simulink model "ActiveBalancerCopy"  (R2021a)
settings: Solver=VariableStepAuto  StartTime=0.0  StopTime=30  RelTol=1e-3
undefined symbols (not defined in the file): Ion, Lithium
libraries: spsIdealSwitchLib x12, spsSeriesRLCBranchLib x12, spsBatteryLib x6, spsDiodeLib x6, spsDCVoltageSourceLib x3, spsGroundLib x3, spsPWMGenerator2LevelLib x3, spspowerguiLib x1
settings Model: Creator=jafar  LastModifiedBy=jafar

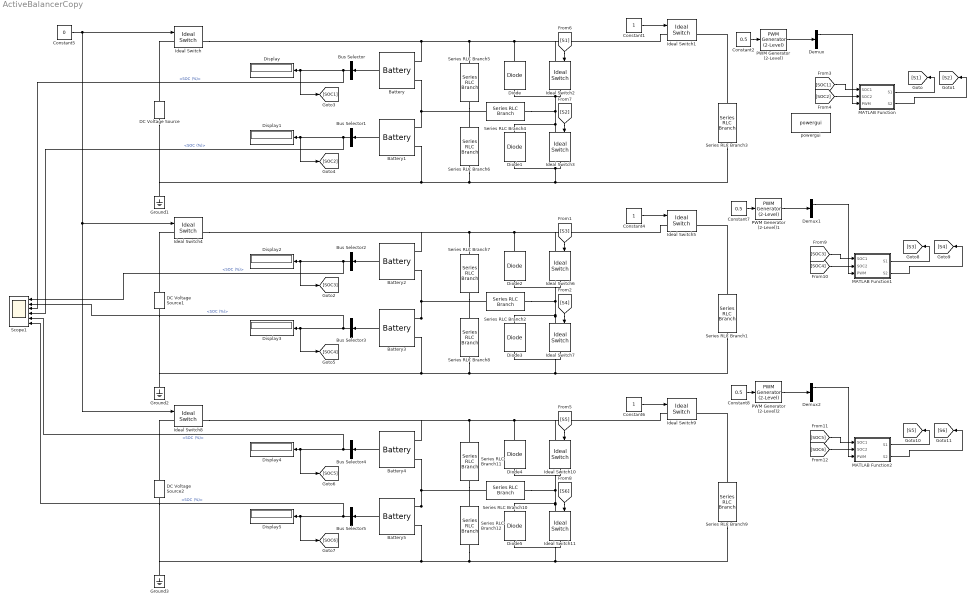
== system ActiveBalancerCopy ==
  Battery : spsBatteryLib/Battery  BatType=Lithium-Ion  ShowTempParam=off  ThermalPreset=no  ShowAgeParam=off  NomV=3.7  NomQ=5.4  SOC=20  Batt_Tr=30  PresetModel=on  MaxQ=5.4  MinV=2.775  FullV=4.3068  Dis_rate=2.3478  R=0.0068519  Normal_OP=4.8835  expZone="[3.9974      0.2653]"  current=[6.5 13 32.5]  Units=Time  Tci=20  NomT=20  T2=-30  MaxQ2=4.8  FullV2=7.1  Normal_OP2=5.655  expZone2="[6.58           1]"  Rca=0.6  ti=2000  Dp=0  Neq0=0  Tsim=1e6  Ta1=25  Qeol=5.4*0.9  Reol=0.013333*1.2  Char_age=[2.3478, 3]  Dis_age=[2.3478, 10]  N1=1500  N2=10500  N3=1000  N4=1400  Ta2=45  N5=950
  Battery1 : spsBatteryLib/Battery  BatType=Lithium-Ion  ShowTempParam=off  ThermalPreset=no  ShowAgeParam=off  NomV=3.7  NomQ=5.4  SOC=30  Batt_Tr=30  PresetModel=on  MaxQ=5.4  MinV=2.775  FullV=4.3068  Dis_rate=2.3478  R=0.0068519  Normal_OP=4.8835  expZone="[3.9974      0.2653]"  current=[6.5 13 32.5]  Units=Time  Tci=20  NomT=20  T2=-30  MaxQ2=4.8  FullV2=7.1  Normal_OP2=5.655  expZone2="[6.58           1]"  Rca=0.6  ti=2000  Dp=0  Neq0=0  Tsim=1e6  Ta1=25  Qeol=5.4*0.9  Reol=0.013333*1.2  Char_age=[2.3478, 3]  Dis_age=[2.3478, 10]  N1=1500  N2=10500  N3=1000  N4=1400  Ta2=45  N5=950
  Battery2 : spsBatteryLib/Battery  BatType=Lithium-Ion  ShowTempParam=off  ThermalPreset=no  ShowAgeParam=off  NomV=3.7  NomQ=5.4  SOC=40  Batt_Tr=30  PresetModel=on  MaxQ=5.4  MinV=2.775  FullV=4.3068  Dis_rate=2.3478  R=0.0068519  Normal_OP=4.8835  expZone="[3.9974      0.2653]"  current=[6.5 13 32.5]  Units=Time  Tci=20  NomT=20  T2=-30  MaxQ2=4.8  FullV2=7.1  Normal_OP2=5.655  expZone2="[6.58           1]"  Rca=0.6  ti=2000  Dp=0  Neq0=0  Tsim=1e6  Ta1=25  Qeol=5.4*0.9  Reol=0.013333*1.2  Char_age=[2.3478, 3]  Dis_age=[2.3478, 10]  N1=1500  N2=10500  N3=1000  N4=1400  Ta2=45  N5=950
  Battery3 : spsBatteryLib/Battery  BatType=Lithium-Ion  ShowTempParam=off  ThermalPreset=no  ShowAgeParam=off  NomV=3.7  NomQ=5.4  SOC=50  Batt_Tr=30  PresetModel=on  MaxQ=5.4  MinV=2.775  FullV=4.3068  Dis_rate=2.3478  R=0.0068519  Normal_OP=4.8835  expZone="[3.9974      0.2653]"  current=[6.5 13 32.5]  Units=Time  Tci=20  NomT=20  T2=-30  MaxQ2=4.8  FullV2=7.1  Normal_OP2=5.655  expZone2="[6.58           1]"  Rca=0.6  ti=2000  Dp=0  Neq0=0  Tsim=1e6  Ta1=25  Qeol=5.4*0.9  Reol=0.013333*1.2  Char_age=[2.3478, 3]  Dis_age=[2.3478, 10]  N1=1500  N2=10500  N3=1000  N4=1400  Ta2=45  N5=950
  Battery4 : spsBatteryLib/Battery  BatType=Lithium-Ion  ShowTempParam=off  ThermalPreset=no  ShowAgeParam=off  NomV=3.7  NomQ=5.4  SOC=60  Batt_Tr=30  PresetModel=on  MaxQ=5.4  MinV=2.775  FullV=4.3068  Dis_rate=2.3478  R=0.0068519  Normal_OP=4.8835  expZone="[3.9974      0.2653]"  current=[6.5 13 32.5]  Units=Time  Tci=20  NomT=20  T2=-30  MaxQ2=4.8  FullV2=7.1  Normal_OP2=5.655  expZone2="[6.58           1]"  Rca=0.6  ti=2000  Dp=0  Neq0=0  Tsim=1e6  Ta1=25  Qeol=5.4*0.9  Reol=0.013333*1.2  Char_age=[2.3478, 3]  Dis_age=[2.3478, 10]  N1=1500  N2=10500  N3=1000  N4=1400  Ta2=45  N5=950
  Battery5 : spsBatteryLib/Battery  BatType=Lithium-Ion  ShowTempParam=off  ThermalPreset=no  ShowAgeParam=off  NomV=3.7  NomQ=5.4  SOC=70  Batt_Tr=30  PresetModel=on  MaxQ=5.4  MinV=2.775  FullV=4.3068  Dis_rate=2.3478  R=0.0068519  Normal_OP=4.8835  expZone="[3.9974      0.2653]"  current=[6.5 13 32.5]  Units=Time  Tci=20  NomT=20  T2=-30  MaxQ2=4.8  FullV2=7.1  Normal_OP2=5.655  expZone2="[6.58           1]"  Rca=0.6  ti=2000  Dp=0  Neq0=0  Tsim=1e6  Ta1=25  Qeol=5.4*0.9  Reol=0.013333*1.2  Char_age=[2.3478, 3]  Dis_age=[2.3478, 10]  N1=1500  N2=10500  N3=1000  N4=1400  Ta2=45  N5=950
  Bus Selector{,1..5} (6 alike) : BusSelector  OutputSignals=SOC (%)
  Constant1 : Constant
  Constant2 : Constant  Value=0.5
  Constant4 : Constant
  Constant5 : Constant  Value=0
  Constant6 : Constant
  Constant7 : Constant  Value=0.5
  Constant8 : Constant  Value=0.5
  DC Voltage Source : spsDCVoltageSourceLib/DC Voltage Source  Amplitude=12  Measurements=None
  DC Voltage Source1 : spsDCVoltageSourceLib/DC Voltage Source  Amplitude=12  Measurements=None
  DC Voltage Source2 : spsDCVoltageSourceLib/DC Voltage Source  Amplitude=12  Measurements=None
  Demux : Demux  Outputs=2
  Demux1 : Demux  Outputs=2
  Demux2 : Demux  Outputs=2
  Diode{,1..5} (6 alike) : spsDiodeLib/Diode  Ron=0.001  Lon=0  Vf=0.8  IC=0  UseSnubber=0  Rs=500  Cs=250e-9  Measurements=off
  Display{,1..5} (6 alike) : Display
  Ground1 : spsGroundLib/Ground  LConnTagsString=a
  Ground2 : spsGroundLib/Ground  LConnTagsString=a
  Ground3 : spsGroundLib/Ground  LConnTagsString=a
  Ideal Switch{,1,4..5,8..9} (6 alike) : spsIdealSwitchLib/Ideal Switch  Ron=0.001  Lon=0  IC=0  Rs=1e5  Cs=inf  Measurements=on
  Ideal Switch{2..3,6..7,10..11} (6 alike) : spsIdealSwitchLib/Ideal Switch  Ron=0.001  Lon=0  IC=0  Rs=1e5  Cs=inf  Measurements=off
  MATLAB Function : MATLAB Function  TreatAsAtomicUnit=on
  MATLAB Function1 : MATLAB Function  TreatAsAtomicUnit=on
  MATLAB Function2 : MATLAB Function  TreatAsAtomicUnit=on
  PWM Generator (2-Level) : spsPWMGenerator2LevelLib/PWM Generator (2-Level)  ModulatorType=Single-phase half-bridge (2 pulses)  ModulatorMode=Unsynchronized  Fc=500  Pc=0  nF=27  MinMax="[ -1  1 ]"  SamplingTechnique=Natural  ModulatingSignals=off  m=0.8  Freq=60  Phase=0  Ts=0  ShowCarrierOutport=off
  PWM Generator (2-Level)1 : spsPWMGenerator2LevelLib/PWM Generator (2-Level)  ModulatorType=Single-phase half-bridge (2 pulses)  ModulatorMode=Unsynchronized  Fc=500  Pc=0  nF=27  MinMax="[ -1  1 ]"  SamplingTechnique=Natural  ModulatingSignals=off  m=0.8  Freq=60  Phase=0  Ts=0  ShowCarrierOutport=off
  PWM Generator (2-Level)2 : spsPWMGenerator2LevelLib/PWM Generator (2-Level)  ModulatorType=Single-phase half-bridge (2 pulses)  ModulatorMode=Unsynchronized  Fc=500  Pc=0  nF=27  MinMax="[ -1  1 ]"  SamplingTechnique=Natural  ModulatingSignals=off  m=0.8  Freq=60  Phase=0  Ts=0  ShowCarrierOutport=off
  Scope1 : Scope  NumInputPorts=6
  Series RLC Branch1 : spsSeriesRLCBranchLib/Series RLC Branch  LConnTagsString=__new0  RConnTagsString=__new0  BranchType=R  Resistance=1  Inductance=1e-3  SetiL0=off  InitialCurrent=0  Capacitance=1e-6  Setx0=off  InitialVoltage=0  Measurements=None
  Series RLC Branch10 : spsSeriesRLCBranchLib/Series RLC Branch  LConnTagsString=__new0  RConnTagsString=__new0  BranchType=L  Resistance=1  Inductance=1e-3  SetiL0=off  InitialCurrent=0  Capacitance=1e-6  Setx0=off  InitialVoltage=0  Measurements=None
  Series RLC Branch{5..8,11..12} (6 alike) : spsSeriesRLCBranchLib/Series RLC Branch  LConnTagsString=__new0  RConnTagsString=__new0  BranchType=C  Resistance=1  Inductance=1e-3  SetiL0=off  InitialCurrent=0  Capacitance=1e-6  Setx0=off  InitialVoltage=0  Measurements=None
  Series RLC Branch2 : spsSeriesRLCBranchLib/Series RLC Branch  LConnTagsString=__new0  RConnTagsString=__new0  BranchType=L  Resistance=1  Inductance=1e-3  SetiL0=off  InitialCurrent=0  Capacitance=1e-6  Setx0=off  InitialVoltage=0  Measurements=None
  Series RLC Branch3 : spsSeriesRLCBranchLib/Series RLC Branch  LConnTagsString=__new0  RConnTagsString=__new0  BranchType=R  Resistance=1  Inductance=1e-3  SetiL0=off  InitialCurrent=0  Capacitance=1e-6  Setx0=off  InitialVoltage=0  Measurements=None
  Series RLC Branch4 : spsSeriesRLCBranchLib/Series RLC Branch  LConnTagsString=__new0  RConnTagsString=__new0  BranchType=L  Resistance=1  Inductance=1e-3  SetiL0=off  InitialCurrent=0  Capacitance=1e-6  Setx0=off  InitialVoltage=0  Measurements=None
  Series RLC Branch9 : spsSeriesRLCBranchLib/Series RLC Branch  LConnTagsString=__new0  RConnTagsString=__new0  BranchType=R  Resistance=1  Inductance=1e-3  SetiL0=off  InitialCurrent=0  Capacitance=1e-6  Setx0=off  InitialVoltage=0  Measurements=None
  powergui : spspowerguiLib/powergui  Priority=1  SimulationMode=Discrete  SampleTime=50e-5  frequency=60  Iterations=50  frequencyindice=0  Pbase=100e6  ErrMax=1e-4  UnitsV=kV  UnitsW=MW  buscounter=0  FunctionMessages=off  echomessages=off  EnableUseOfTLC=off  CurrentSourceSwitches=off  DisableSnubberDevices=off  DisableRonSwitches=off  DisableVfSwitches=off  DisplayEquations=off  AutomaticDiscreteSolvers=off  SolverType=Tustin/Backward Euler (TBE)  Interpol=off  ExternalGateDelay=off  methode=off  Ts=100  x0status=blocks  SPID=on  SwTol=0  HookPort=off  NonlinearTolerance=1e-4  nMaxIteration=100  ContinueOnMaxIteration=off  RestoreLinks=warning  ResistiveCurrentMeasurement=off  Frange=[0:2:500]  Ylog=off  Xlog=on  ShowGrid=off  save=off  variable=ZData  structure=0  ZoomFFT=off  StartTime=0.0  cycles=1  DisplayStyle=1  fundamental=60  FreqAxis=off  MaxFrequency=1000  frequencyindicesteady=1  RmsSteady=1  display=off
  wires:
  [SOC1] -> MATLAB Function/1(SOC1)
  [SOC2] -> MATLAB Function/2(SOC2)
  Constant5/1 -> Ideal Switch/1, Ideal Switch4/1, Ideal Switch8/1
  MATLAB Function/1(S1) -> [S1]
  Battery/1 -> Bus Selector/1
  Bus Selector1/1 -> Scope1/4, [SOC2], Display1/1  "<SOC (%)>"
  Battery1/1 -> Bus Selector1/1
  MATLAB Function/2(S2) -> [S2]
  Constant1/1 -> Ideal Switch1/1
  Bus Selector/1 -> Scope1/3, [SOC1], Display/1  "<SOC (%)>"
  [S1] -> Ideal Switch2/1
  [S2] -> Ideal Switch3/1
  Constant2/1 -> PWM Generator (2-Level)/1
  PWM Generator (2-Level)/1 -> Demux/1
  Demux/1 -> MATLAB Function/3(PWM)
  Battery3/1 -> Bus Selector3/1
  Bus Selector3/1 -> Scope1/2, [SOC4], Display3/1  "<SOC (%)>"
  Bus Selector2/1 -> Scope1/1, [SOC3], Display2/1  "<SOC (%)>"
  [S3] -> Ideal Switch6/1
  [S4] -> Ideal Switch7/1
  Battery2/1 -> Bus Selector2/1
  Constant4/1 -> Ideal Switch5/1
  Battery5/1 -> Bus Selector5/1
  Bus Selector5/1 -> Scope1/6, [SOC6], Display5/1  "<SOC (%)>"
  Bus Selector4/1 -> Scope1/5, [SOC5], Display4/1  "<SOC (%)>"
  [S5] -> Ideal Switch10/1
  [S6] -> Ideal Switch11/1
  Battery4/1 -> Bus Selector4/1
  Constant6/1 -> Ideal Switch9/1
  Constant7/1 -> PWM Generator (2-Level)1/1
  Demux1/1 -> MATLAB Function1/3(PWM)
  [SOC4] -> MATLAB Function1/2(SOC2)
  MATLAB Function1/2(S2) -> [S4]
  MATLAB Function1/1(S1) -> [S3]
  PWM Generator (2-Level)1/1 -> Demux1/1
  [SOC3] -> MATLAB Function1/1(SOC1)
  Constant8/1 -> PWM Generator (2-Level)2/1
  Demux2/1 -> MATLAB Function2/3(PWM)
  [SOC6] -> MATLAB Function2/2(SOC2)
  MATLAB Function2/2(S2) -> [S6]
  MATLAB Function2/1(S1) -> [S5]
  PWM Generator (2-Level)2/1 -> Demux2/1
  [SOC5] -> MATLAB Function2/1(SOC1)
  connections:
  Ideal Switch3/RConn1 -- Series RLC Branch3/RConn1 -- Ground1/LConn1 -- DC Voltage Source/LConn1 -- Battery1/LConn2 -- Series RLC Branch6/RConn1 -- Diode1/LConn1
  Battery/LConn2 -- Series RLC Branch6/LConn1 -- Series RLC Branch5/RConn1 -- Series RLC Branch4/LConn1 -- Battery1/LConn1
  Battery/LConn1 -- Ideal Switch/RConn1 -- Series RLC Branch5/LConn1 -- Ideal Switch2/LConn1 -- Ideal Switch1/LConn1 -- Diode/RConn1
  Series RLC Branch3/LConn1 -- Ideal Switch1/RConn1
  Ideal Switch/LConn1 -- DC Voltage Source/RConn1
  Ideal Switch2/RConn1 -- Series RLC Branch4/RConn1 -- Diode1/RConn1 -- Ideal Switch3/LConn1 -- Diode/LConn1
  Ideal Switch7/LConn1 -- Ideal Switch6/RConn1 -- Diode2/LConn1 -- Series RLC Branch2/RConn1 -- Diode3/RConn1
  Battery3/LConn1 -- Battery2/LConn2 -- Series RLC Branch8/LConn1 -- Series RLC Branch7/RConn1 -- Series RLC Branch2/LConn1
  Series RLC Branch8/RConn1 -- Ideal Switch7/RConn1 -- Diode3/LConn1 -- Series RLC Branch1/RConn1 -- Ground2/LConn1 -- DC Voltage Source1/LConn1 -- Battery3/LConn2
  Diode2/RConn1 -- Battery2/LConn1 -- Ideal Switch4/RConn1 -- Series RLC Branch7/LConn1 -- Ideal Switch6/LConn1 -- Ideal Switch5/LConn1
  Series RLC Branch1/LConn1 -- Ideal Switch5/RConn1
  Ideal Switch4/LConn1 -- DC Voltage Source1/RConn1
  Ideal Switch11/LConn1 -- Ideal Switch10/RConn1 -- Diode4/LConn1 -- Series RLC Branch10/RConn1 -- Diode5/RConn1
  Battery5/LConn1 -- Battery4/LConn2 -- Series RLC Branch12/LConn1 -- Series RLC Branch11/RConn1 -- Series RLC Branch10/LConn1
  Series RLC Branch12/RConn1 -- Ideal Switch11/RConn1 -- Diode5/LConn1 -- Series RLC Branch9/RConn1 -- Ground3/LConn1 -- DC Voltage Source2/LConn1 -- Battery5/LConn2
  Diode4/RConn1 -- Battery4/LConn1 -- Ideal Switch8/RConn1 -- Series RLC Branch11/LConn1 -- Ideal Switch10/LConn1 -- Ideal Switch9/LConn1
  Series RLC Branch9/LConn1 -- Ideal Switch9/RConn1
  Ideal Switch8/LConn1 -- DC Voltage Source2/RConn1

== matlab function ActiveBalancerCopy/MATLAB Function1 ==
  data: SOC1 input; S1 output; SOC2 input; S2 output; PWM input
function [S1,S2] = fcn(SOC1,SOC2,PWM)

if SOC2<SOC1
    S1 = PWM;
    S2 = 0;
elseif SOC1<SOC2
    S1 = 0;
    S2 = PWM;
else
    S1 = 0;
    S2 = 0;
end

== matlab function ActiveBalancerCopy/MATLAB Function ==
  data: SOC1 input; S1 output; SOC2 input; S2 output; PWM input
function [S1,S2] = fcn(SOC1,SOC2,PWM)

if SOC2<SOC1
    S1 = PWM;
    S2 = 0;
elseif SOC1<SOC2
    S1 = 0;
    S2 = PWM;
else
    S1 = 0;
    S2 = 0;
end

== matlab function ActiveBalancerCopy/MATLAB Function2 ==
  data: SOC1 input; S1 output; SOC2 input; S2 output; PWM input
function [S1,S2] = fcn(SOC1,SOC2,PWM)

if SOC2<SOC1
    S1 = PWM;
    S2 = 0;
elseif SOC1<SOC2
    S1 = 0;
    S2 = PWM;
else
    S1 = 0;
    S2 = 0;
end
